simulink model "lab1handson"  (R2020a)
settings: Solver=VariableStepAuto  StartTime=0.0  StopTime=10.0  RelTol=1e-3
values from neighbouring files (symbols this model uses):
  a = -3    [matlab.mat]    (also in matlab2.mat)
  b = -4    [matlab.mat]    (also in matlab2.mat)
  Ki = 4    [matlab.mat]    (also in matlab2.mat)
  Kp = 36    [matlab.mat]    (also in matlab2.mat)
  m = 25    [matlab.mat]    (also in matlab2.mat)
  Ts = 0.01    [matlab.mat]    (also in matlab2.mat)
settings Model: Creator=pawankumarf  LastModifiedBy=pawankumarf
settings DataIOCC: ExternalInput=[t, stin]  LoadExternalInput=on  SaveFormat=Array  ReturnWorkspaceOutputs=off

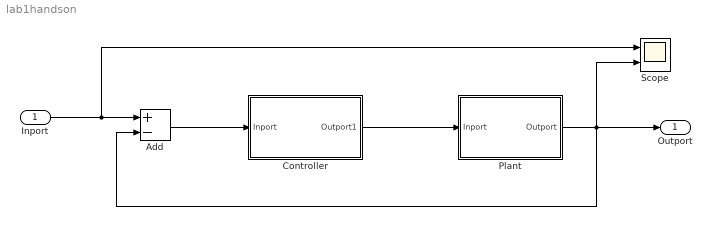
== system lab1handson ==
  Inport : Inport
  Add : Sum  Inputs=+-
  Controller : Subsystem
  Plant : Subsystem
  Scope : Scope  NumInputPorts=2
  Outport : Outport
  wires:
  Controller/1(Outport1) -> Plant/1(Inport)
  Plant/1(Outport) -> Scope/2, Outport/1, Add/2
  Add/1 -> Controller/1(Inport)
  Inport/1 -> Scope/1, Add/1

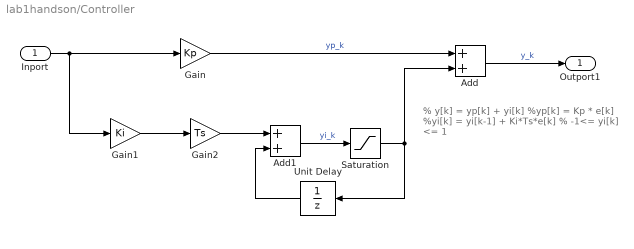
== system lab1handson/Controller ==
  note: % y[k] = yp[k] + yi[k]
      | %yp[k] = Kp * e[k]
      | %yi[k] = yi[k-1] + Ki*Ts*e[k]
      | % -1<= yi[k] <= 1
  Inport : Inport
  Add : Sum
  Add1 : Sum
  Gain : Gain  Gain=Kp
  Gain1 : Gain  Gain=Ki
  Gain2 : Gain  Gain=Ts
  Saturation : Saturate  UpperLimit=1  LowerLimit=-1
  Unit Delay : UnitDelay  SampleTime=-1  HasFrameUpgradeWarning=on
  Outport1 : Outport
  wires:
  Gain/1 -> Add/1  "yp_k"
  Gain2/1 -> Add1/1
  Add/1 -> Outport1/1  "y_k"
  Inport/1 -> Gain1/1, Gain/1
  Gain1/1 -> Gain2/1
  Unit Delay/1 -> Add1/2
  Saturation/1 -> Add/2, Unit Delay/1
  Add1/1 -> Saturation/1  "yi_k"

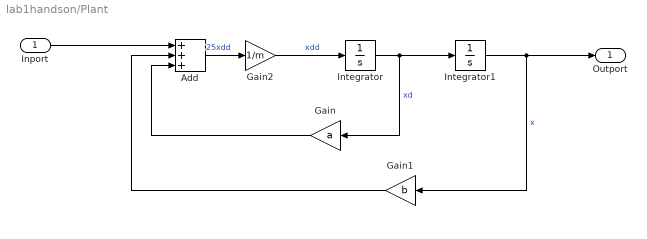
== system lab1handson/Plant ==
  Inport : Inport
  Add : Sum  Inputs=+++
  Gain : Gain  Gain=a
  Gain1 : Gain  Gain=b
  Gain2 : Gain  Gain=1/m
  Integrator : Integrator
  Integrator1 : Integrator
  Outport : Outport
  wires:
  Integrator/1 -> Integrator1/1, Gain/1  "xd"
  Gain1/1 -> Add/2
  Add/1 -> Gain2/1  "25xdd"
  Gain/1 -> Add/3
  Gain2/1 -> Integrator/1  "xdd"
  Integrator1/1 -> Outport/1, Gain1/1  "x"
  Inport/1 -> Add/1
